simulink model "TriggeredSubsystems"  (R2012b)
settings: Solver=ode45  SolverMode=SingleTasking  StartTime=0.0  StopTime=10.0  RelTol=1e-3
settings Model: Creator=odj  LastModifiedBy=TSR2
settings DataIOCC: SignalLoggingSaveFormat=ModelDataLogs
settings OptimizationCC: BlockReduction=off  BooleanDataType=off
settings DebuggingCC: SaveWithParameterizedLinksMsg=none  SignalResolutionControl=TryResolveAllWithWarning  SolverPrmCheckMsg=none  MultiTaskDSMMsg=warning  MultiTaskCondExecSysMsg=none  StrictBusMsg=None
settings HardwareCC: TargetIntDivRoundTo=Zero  TargetEndianess=LittleEndian  TargetHWDeviceType=MATLAB Host  ProdEqTarget=off
settings RTWCC: SystemTargetFile=rtwsfcnfmi.tlc  TemplateMakefile=rtwsfcnfmi_tmf  Description=S-Function Target with Functional Mockup Interface (FMI)  ProcessScript=rtwsfcnfmi_make_rtw_hook  IncludeERTFirstTime=on
settings STFCustomTargetCC: CodeReplacementLibrary=ANSI_C  ModelReferenceCompliant=off  CompOptLevelCompliant=on  GeneratePreprocessorConditionals=Disable all  SystemTargetFile=rtwsfcnfmi.tlc

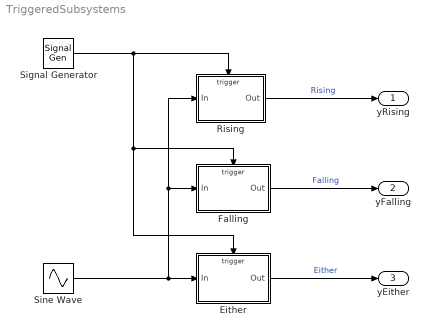
== system TriggeredSubsystems ==
  Either : Subsystem
  Falling : Subsystem
  Rising : Subsystem
  Signal Generator : SignalGenerator  WaveForm=square  Amplitude=0.5
  Sine Wave : Sin  Frequency=8  SampleTime=0
  yRising : Outport
  yFalling : Outport  Port=2
  yEither : Outport  Port=3
  wires:
  Signal Generator/1 -> Rising/Trigger, Either/Trigger, Falling/Trigger
  Sine Wave/1 -> Falling/1(In), Rising/1(In), Either/1(In)
  Rising/1(Out) -> yRising/1  "Rising"
  Falling/1(Out) -> yFalling/1  "Falling"
  Either/1(Out) -> yEither/1  "Either"

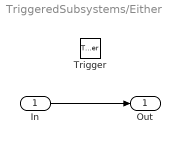
== system TriggeredSubsystems/Either ==
  In : Inport
  Trigger : TriggerPort  TriggerType=either
  Out : Outport  InitialOutput=0
  wires:
  In/1 -> Out/1

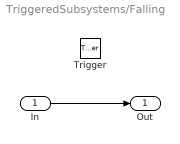
== system TriggeredSubsystems/Falling ==
  In : Inport
  Trigger : TriggerPort  TriggerType=falling
  Out : Outport  InitialOutput=0
  wires:
  In/1 -> Out/1

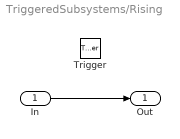
== system TriggeredSubsystems/Rising ==
  In : Inport
  Trigger : TriggerPort
  Out : Outport  InitialOutput=0
  wires:
  In/1 -> Out/1
